simulink model "WelcomeBkwdStEnCtrl"  (R2018b)
settings: Solver=FixedStepDiscrete  StartTime=0.0  StopTime=10.0  FixedStep=0.01  RelTol=1e-3
undefined symbols (not defined in the file or in its folder): data, SecRwLtStBkReclnEn_Clear, SecRwLtStBkReclnEn_Set, SecRwLtStFwdBkwdEn_Clear, SecRwLtStFwdBkwdEn_Set, SecRwLtStHdrstFwdBkwdEn_Clear, SecRwLtStHdrstFwdBkwdEn_Set, SecRwLtStHdrstUpwdDnwdEn_Clear, SecRwLtStHdrstUpwdDnwdEn_Set, SecRwRtStBkReclnEn_Clear, SecRwRtStBkReclnEn_Set, SecRwRtStFwdBkwdEn_Clear, SecRwRtStFwdBkwdEn_Set, SecRwRtStHdrstFwdBkwdEn_Clear, SecRwRtStHdrstFwdBkwdEn_Set, SecRwRtStHdrstUpwdDnwdEn_Clear, SecRwRtStHdrstUpwdDnwdEn_Set
libraries: simulink x1
settings Model: ModifiedHistory=2023.8.1 V2.0.0 CR421790 增加模式21-26  Creator=sn2xws  LastModifiedBy=sn2xws
settings DataIOCC: SaveFormat=StructureWithTime
settings OptimizationCC: DefaultParameterBehavior=Inlined  EnhancedBackFolding=on  PassReuseOutputArgsAs=Individual arguments  ZeroExternalMemoryAtStartup=off  ZeroInternalMemoryAtStartup=off  OptimizeBlockOrder=speed  DifferentSizesBufferReuse=on  OptimizationCustomize=off
settings DebuggingCC: ParameterTunabilityLossMsg=error
settings SFSimCC: MATLABDynamicMemAlloc=off
settings RTWCC: SystemTargetFile=autosar.tlc  GenCodeOnly=on  TemplateMakefile=ert_default_tmf  Description=AUTOSAR  GenerateReport=on  IncludeHyperlinkInReport=on  LaunchReport=on  GenerateTraceInfo=on  GenerateTraceReport=on  GenerateTraceReportSl=on  GenerateTraceReportSf=on  GenerateTraceReportEml=on  GenerateCodeMetricsReport=on
settings CodeAppCC: ForceParamTrailComments=on  IgnoreCustomStorageClasses=off  OperatorAnnotations=on  SimulinkDataObjDesc=on  SFDataObjDesc=on  InsertBlockDesc=on
settings STFCustomTargetCC: TargetLangStandard=C99 (ISO)  MultiwordLength=256  ParMdlRefBuildCompliant=on  CompOptLevelCompliant=on  IncludeMdlTerminateFcn=off  CombineOutputUpdateFcns=on  SuppressErrorStatus=on  ERTCustomFileBanners=on  SupportNonFinite=off  SupportComplex=off  SupportContinuousTime=off  SupportNonInlinedSFcns=off  RemoveResetFunc=on  MATLABClassNameForMDSCustomization=Simulink.SoftwareTarget.ERTCustomization  AutosarCompliant=on  UseToolchainInfoCompliant=on  LookupTableObjectStructAxisOrder=2,1,3,4,...  LUTObjectStructOrderEvenSpacing=Size,Table,Breakpoints  SystemTargetFile=autosar.tlc
settings ERTTargetCC: TargetLangStandard=C99 (ISO)  ConcurrentExecutionCompliant=off  IncludeMdlTerminateFcn=off  SuppressErrorStatus=on  SupportNonFinite=off  SupportComplex=off  ModelStepFunctionPrototypeControlCompliant=off  CPPClassGenCompliant=off  AutosarCompliant=on  LookupTableObjectStructAxisOrder=2,1,3,4,...  LUTObjectStructOrderEvenSpacing=Size,Table,Breakpoints  InlinedParameterPlacement=NonHierarchical  ERTCustomFileTemplate=example_file_process.tlc  ERTFilePackagingFormat=Compact

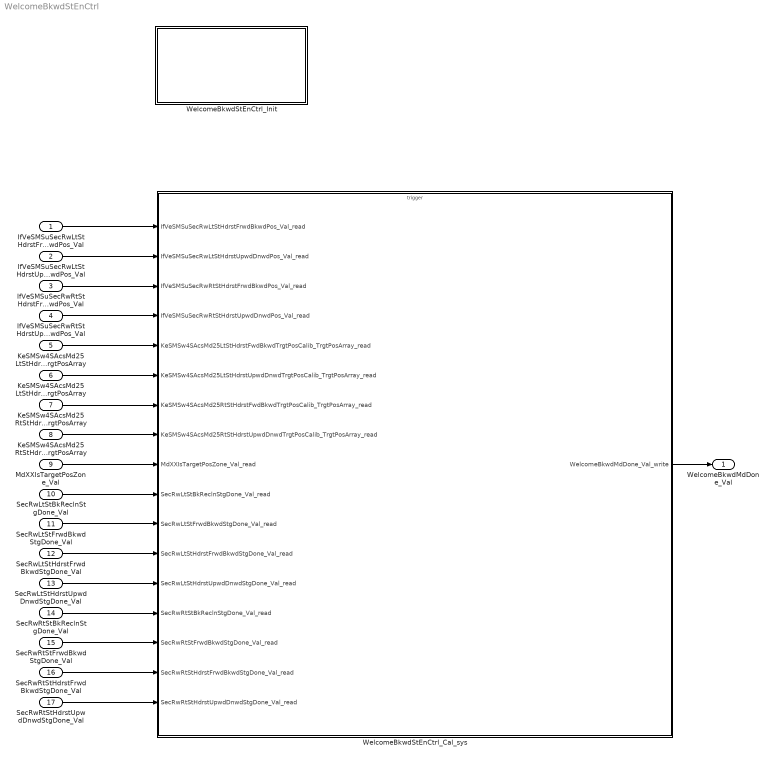
== system WelcomeBkwdStEnCtrl ==
  IfVeSMSuSecRwLtStHdrstFrwdBkwdPos_Val : Inport  OutDataTypeStr=uint16  PortDimensions=1
  IfVeSMSuSecRwLtStHdrstUpwdDnwdPos_Val : Inport  Port=2  OutDataTypeStr=uint16  PortDimensions=1
  IfVeSMSuSecRwRtStHdrstFrwdBkwdPos_Val : Inport  Port=3  OutDataTypeStr=uint16  PortDimensions=1
  IfVeSMSuSecRwRtStHdrstUpwdDnwdPos_Val : Inport  Port=4  OutDataTypeStr=uint16  PortDimensions=1
  KeSMSw4SAcsMd25LtStHdrstFwdBkwdTrgtPosCalib_TrgtPosArray : Inport  Description=|  Port=5  OutDataTypeStr=uint16  PortDimensions=3
      | 0:Pos
      | 1:Max
      | 2:Min
  KeSMSw4SAcsMd25LtStHdrstUpwdDnwdTrgtPosCalib_TrgtPosArray : Inport  Description=|  Port=6  OutDataTypeStr=uint16  PortDimensions=3
      | 0:Pos
      | 1:Max
      | 2:Min
  KeSMSw4SAcsMd25RtStHdrstFwdBkwdTrgtPosCalib_TrgtPosArray : Inport  Description=|  Port=7  OutDataTypeStr=uint16  PortDimensions=3
      | 0:Pos
      | 1:Max
      | 2:Min
  KeSMSw4SAcsMd25RtStHdrstUpwdDnwdTrgtPosCalib_TrgtPosArray : Inport  Description=|  Port=8  OutDataTypeStr=uint16  PortDimensions=3
      | 0:Pos
      | 1:Max
      | 2:Min
  MdXXIsTargetPosZone_Val : Inport  Port=9  OutDataTypeStr=uint32  PortDimensions=1
  SecRwLtStBkReclnStgDone_Val : Inport  Port=10  OutDataTypeStr=boolean  PortDimensions=1
  SecRwLtStFrwdBkwdStgDone_Val : Inport  Port=11  OutDataTypeStr=boolean  PortDimensions=1
  SecRwLtStHdrstFrwdBkwdStgDone_Val : Inport  Port=12  OutDataTypeStr=boolean  PortDimensions=1
  SecRwLtStHdrstUpwdDnwdStgDone_Val : Inport  Port=13  OutDataTypeStr=boolean  PortDimensions=1
  SecRwRtStBkReclnStgDone_Val : Inport  Port=14  OutDataTypeStr=boolean  PortDimensions=1
  SecRwRtStFrwdBkwdStgDone_Val : Inport  Port=15  OutDataTypeStr=boolean  PortDimensions=1
  SecRwRtStHdrstFrwdBkwdStgDone_Val : Inport  Port=16  OutDataTypeStr=boolean  PortDimensions=1
  SecRwRtStHdrstUpwdDnwdStgDone_Val : Inport  Port=17  OutDataTypeStr=boolean  PortDimensions=1
  WelcomeBkwdStEnCtrl_Cal_sys : Subsystem
  WelcomeBkwdStEnCtrl_Init : Subsystem
  WelcomeBkwdMdDone_Val : Outport  OutDataTypeStr=uint8  PortDimensions=1
  wires:
  IfVeSMSuSecRwLtStHdrstFrwdBkwdPos_Val/1 -> WelcomeBkwdStEnCtrl_Cal_sys/1(IfVeSMSuSecRwLtStHdrstFrwdBkwdPos_Val_read)
  IfVeSMSuSecRwLtStHdrstUpwdDnwdPos_Val/1 -> WelcomeBkwdStEnCtrl_Cal_sys/2(IfVeSMSuSecRwLtStHdrstUpwdDnwdPos_Val_read)
  IfVeSMSuSecRwRtStHdrstFrwdBkwdPos_Val/1 -> WelcomeBkwdStEnCtrl_Cal_sys/3(IfVeSMSuSecRwRtStHdrstFrwdBkwdPos_Val_read)
  IfVeSMSuSecRwRtStHdrstUpwdDnwdPos_Val/1 -> WelcomeBkwdStEnCtrl_Cal_sys/4(IfVeSMSuSecRwRtStHdrstUpwdDnwdPos_Val_read)
  KeSMSw4SAcsMd25LtStHdrstFwdBkwdTrgtPosCalib_TrgtPosArray/1 -> WelcomeBkwdStEnCtrl_Cal_sys/5(KeSMSw4SAcsMd25LtStHdrstFwdBkwdTrgtPosCalib_TrgtPosArray_read)
  KeSMSw4SAcsMd25LtStHdrstUpwdDnwdTrgtPosCalib_TrgtPosArray/1 -> WelcomeBkwdStEnCtrl_Cal_sys/6(KeSMSw4SAcsMd25LtStHdrstUpwdDnwdTrgtPosCalib_TrgtPosArray_read)
  KeSMSw4SAcsMd25RtStHdrstFwdBkwdTrgtPosCalib_TrgtPosArray/1 -> WelcomeBkwdStEnCtrl_Cal_sys/7(KeSMSw4SAcsMd25RtStHdrstFwdBkwdTrgtPosCalib_TrgtPosArray_read)
  KeSMSw4SAcsMd25RtStHdrstUpwdDnwdTrgtPosCalib_TrgtPosArray/1 -> WelcomeBkwdStEnCtrl_Cal_sys/8(KeSMSw4SAcsMd25RtStHdrstUpwdDnwdTrgtPosCalib_TrgtPosArray_read)
  MdXXIsTargetPosZone_Val/1 -> WelcomeBkwdStEnCtrl_Cal_sys/9(MdXXIsTargetPosZone_Val_read)
  SecRwLtStBkReclnStgDone_Val/1 -> WelcomeBkwdStEnCtrl_Cal_sys/10(SecRwLtStBkReclnStgDone_Val_read)
  SecRwLtStFrwdBkwdStgDone_Val/1 -> WelcomeBkwdStEnCtrl_Cal_sys/11(SecRwLtStFrwdBkwdStgDone_Val_read)
  SecRwLtStHdrstFrwdBkwdStgDone_Val/1 -> WelcomeBkwdStEnCtrl_Cal_sys/12(SecRwLtStHdrstFrwdBkwdStgDone_Val_read)
  SecRwLtStHdrstUpwdDnwdStgDone_Val/1 -> WelcomeBkwdStEnCtrl_Cal_sys/13(SecRwLtStHdrstUpwdDnwdStgDone_Val_read)
  SecRwRtStBkReclnStgDone_Val/1 -> WelcomeBkwdStEnCtrl_Cal_sys/14(SecRwRtStBkReclnStgDone_Val_read)
  SecRwRtStFrwdBkwdStgDone_Val/1 -> WelcomeBkwdStEnCtrl_Cal_sys/15(SecRwRtStFrwdBkwdStgDone_Val_read)
  SecRwRtStHdrstFrwdBkwdStgDone_Val/1 -> WelcomeBkwdStEnCtrl_Cal_sys/16(SecRwRtStHdrstFrwdBkwdStgDone_Val_read)
  SecRwRtStHdrstUpwdDnwdStgDone_Val/1 -> WelcomeBkwdStEnCtrl_Cal_sys/17(SecRwRtStHdrstUpwdDnwdStgDone_Val_read)
  WelcomeBkwdStEnCtrl_Cal_sys/1(WelcomeBkwdMdDone_Val_write) -> WelcomeBkwdMdDone_Val/1

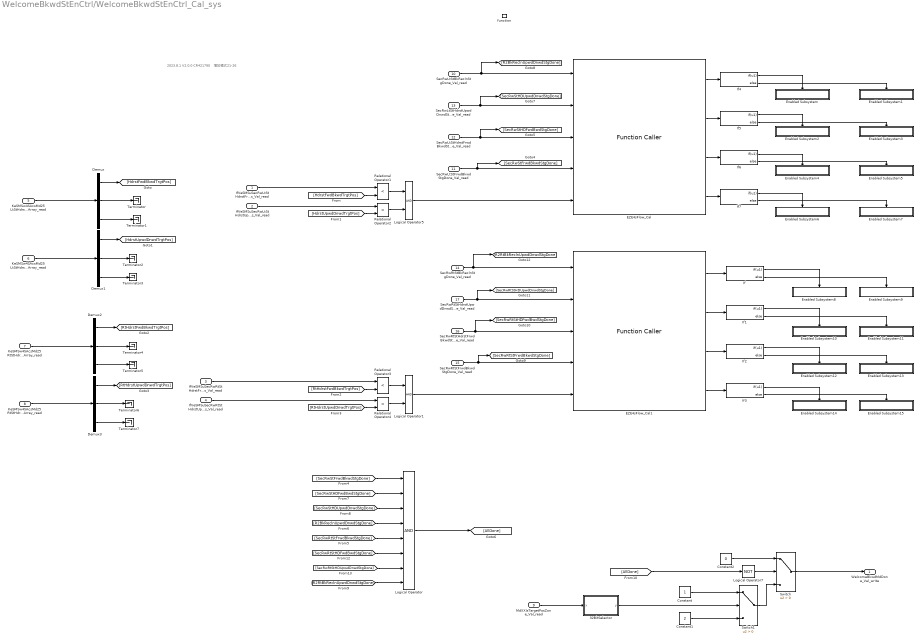
== system WelcomeBkwdStEnCtrl/WelcomeBkwdStEnCtrl_Cal_sys ==
  note: 2023.8.1 V2.0.0 CR421790 增加模式21-26
  IfVeSMSuSecRwLtStHdrstFrwdBkwdPos_Val_read : Inport
  IfVeSMSuSecRwLtStHdrstUpwdDnwdPos_Val_read : Inport  Port=2
  IfVeSMSuSecRwRtStHdrstFrwdBkwdPos_Val_read : Inport  Port=3
  IfVeSMSuSecRwRtStHdrstUpwdDnwdPos_Val_read : Inport  Port=4
  KeSMSw4SAcsMd25LtStHdrstFwdBkwdTrgtPosCalib_TrgtPosArray_read : Inport  Port=5
  KeSMSw4SAcsMd25LtStHdrstUpwdDnwdTrgtPosCalib_TrgtPosArray_read : Inport  Port=6
  KeSMSw4SAcsMd25RtStHdrstFwdBkwdTrgtPosCalib_TrgtPosArray_read : Inport  Port=7
  KeSMSw4SAcsMd25RtStHdrstUpwdDnwdTrgtPosCalib_TrgtPosArray_read : Inport  Port=8
  MdXXIsTargetPosZone_Val_read : Inport  Port=9
  SecRwLtStBkReclnStgDone_Val_read : Inport  Port=10
  SecRwLtStFrwdBkwdStgDone_Val_read : Inport  Port=11
  SecRwLtStHdrstFrwdBkwdStgDone_Val_read : Inport  Port=12
  SecRwLtStHdrstUpwdDnwdStgDone_Val_read : Inport  Port=13
  SecRwRtStBkReclnStgDone_Val_read : Inport  Port=14
  SecRwRtStFrwdBkwdStgDone_Val_read : Inport  Port=15
  SecRwRtStHdrstFrwdBkwdStgDone_Val_read : Inport  Port=16
  SecRwRtStHdrstUpwdDnwdStgDone_Val_read : Inport  Port=17
  function : TriggerPort  TriggerType=function-call  IsSimulinkFunction=on  FunctionName=WelcomeBkwdStEnCtrl_Cal  VariantControl=(inherit)
  32BitSelector : Subsystem  mask(32 Bit Selector){BitNum=24}
      mask prompts: BitNum "Select Bit Number"
      mask help: Allows selection of a particular bit (0-31) out of a packed word up to 32 bits long. Output will be true if the bit number selected via the mask parameter is equal to one.
      mask TypeOptions BitNum: 0 | 1 | 2 | 3 | 4 | 5 | 6 | 7 | 8 | 9 | 10 | 11 | 12 | 13 | 14 | 15 | 16 | 17 | 18 | 19 | 20 | 21 | 22 | 23 | 24 | 25 | 26 | 27 | 28 | 29 | 30 | 31
      mask Display:
      | text(0.5, 0.8,'BIT','horizontalAlignment','center')
      | text(0.5, 0.5,'SELECTOR','horizontalAlignment','center')
      | text(0.5, 0.2,['-- Bit ',char(get_param(gcb,'BitNum')),' --'],'horizontalAlignment','center')
  Constant : Constant  OutDataTypeStr=uint8
  Constant1 : Constant  Value=2  OutDataTypeStr=uint8
  Constant2 : Constant  Value=0  OutDataTypeStr=uint8
  Demux{,1..3} (4 alike) : Demux  Outputs=3
  EZE4sFlow_Cal : FunctionCaller  FunctionPrototype=[BkReclnEn,HdrstUpwdEn,HdrstFrwdEn,SecRwStFrwdBkwdEn] = EZE4sFlow_Cal(BkReclnStgDone,HdrstUpwdDnwdStgDone,HdrstFrwdBkwdStgDone,SecRwStFrwdBkwdStgDone,Chkhdflg)  InputArgumentSpecifications=boolean(true), boolean(true), boolean(true), boolean(true), boolean(true)  OutputArgumentSpecifications=boolean(true), boolean(true), boolean(true), boolean(true)
  EZE4sFlow_Cal1 : FunctionCaller  FunctionPrototype=[BkReclnEn,HdrstUpwdEn,HdrstFrwdEn,SecRwStFrwdBkwdEn] = EZE4sFlow_Cal(BkReclnStgDone,HdrstUpwdDnwdStgDone,HdrstFrwdBkwdStgDone,SecRwStFrwdBkwdStgDone,Chkhdflg)  InputArgumentSpecifications=boolean(true), boolean(true), boolean(true), boolean(true), boolean(true)  OutputArgumentSpecifications=boolean(true), boolean(true), boolean(true), boolean(true)
  Enabled Subsystem : Subsystem  TreatAsAtomicUnit=on
  Enabled Subsystem1 : Subsystem  TreatAsAtomicUnit=on
  Enabled Subsystem10 : Subsystem  TreatAsAtomicUnit=on
  Enabled Subsystem11 : Subsystem  TreatAsAtomicUnit=on
  Enabled Subsystem12 : Subsystem  TreatAsAtomicUnit=on
  Enabled Subsystem13 : Subsystem  TreatAsAtomicUnit=on
  Enabled Subsystem14 : Subsystem  TreatAsAtomicUnit=on
  Enabled Subsystem15 : Subsystem  TreatAsAtomicUnit=on
  Enabled Subsystem2 : Subsystem  TreatAsAtomicUnit=on
  Enabled Subsystem3 : Subsystem  TreatAsAtomicUnit=on
  Enabled Subsystem4 : Subsystem  TreatAsAtomicUnit=on
  Enabled Subsystem5 : Subsystem  TreatAsAtomicUnit=on
  Enabled Subsystem6 : Subsystem  TreatAsAtomicUnit=on
  Enabled Subsystem7 : Subsystem  TreatAsAtomicUnit=on
  Enabled Subsystem8 : Subsystem  TreatAsAtomicUnit=on
  Enabled Subsystem9 : Subsystem  TreatAsAtomicUnit=on
  If{,1..7} (8 alike) : If  IfExpression=u1
  Logical Operator : Logic  Inputs=8  AllPortsSameDT=off  OutDataTypeStr=boolean
  Logical Operator1 : Logic  AllPortsSameDT=off  OutDataTypeStr=boolean
  Logical Operator5 : Logic  AllPortsSameDT=off  OutDataTypeStr=boolean
  Logical Operator7 : Logic  Operator=NOT  AllPortsSameDT=off  OutDataTypeStr=boolean
  Relational Operator{1..4} (4 alike) : RelationalOperator  Operator=<  OutDataTypeStr=boolean  RndMeth=Simplest
  Switch : Switch  Criteria=u2 > Threshold
  Switch1 : Switch  Criteria=u2 > Threshold
  Terminator{,1..7} (8 alike) : Terminator
  WelcomeBkwdMdDone_Val_write : Outport
      settings: EnsureOutportIsVirtual=on
  wires:
  SecRwLtStFrwdBkwdStgDone_Val_read/1 -> EZE4sFlow_Cal/4, [SecRwStFrwdBkwdStgDone]
  SecRwLtStHdrstFrwdBkwdStgDone_Val_read/1 -> [SecRwStHDFwdBwdStgDone], EZE4sFlow_Cal/3
  SecRwLtStHdrstUpwdDnwdStgDone_Val_read/1 -> [SecRwStHDUpwdDnwdStgDone], EZE4sFlow_Cal/2
  SecRwLtStBkReclnStgDone_Val_read/1 -> [R2BkReclnUpwdDnwdStgDone], EZE4sFlow_Cal/1
  SecRwRtStBkReclnStgDone_Val_read/1 -> [R2RtBkReclnUpwdDnwdStgDone], EZE4sFlow_Cal1/1
  SecRwRtStFrwdBkwdStgDone_Val_read/1 -> [SecRwRtStFrwdBkwdStgDone], EZE4sFlow_Cal1/4
  SecRwRtStHdrstFrwdBkwdStgDone_Val_read/1 -> [SecRwRtStHDFwdBwdStgDone], EZE4sFlow_Cal1/3
  SecRwRtStHdrstUpwdDnwdStgDone_Val_read/1 -> [SecRwRtStHDUpwdDnwdStgDone], EZE4sFlow_Cal1/2
  [HdrstFwdBkwdTrgtPos] -> Relational Operator1/2
  IfVeSMSuSecRwLtStHdrstFrwdBkwdPos_Val_read/1 -> Relational Operator1/1
  IfVeSMSuSecRwLtStHdrstUpwdDnwdPos_Val_read/1 -> Relational Operator2/1
  Relational Operator2/1 -> Logical Operator5/2
  [HdrstUpwdDnwdTrgtPos] -> Relational Operator2/2
  Relational Operator1/1 -> Logical Operator5/1
  Logical Operator5/1 -> EZE4sFlow_Cal/5
  Logical Operator1/1 -> EZE4sFlow_Cal1/5
  Relational Operator3/1 -> Logical Operator1/1
  [RtHdrstUpwdDnwdTrgtPos] -> Relational Operator4/2
  Relational Operator4/1 -> Logical Operator1/2
  IfVeSMSuSecRwRtStHdrstUpwdDnwdPos_Val_read/1 -> Relational Operator4/1
  IfVeSMSuSecRwRtStHdrstFrwdBkwdPos_Val_read/1 -> Relational Operator3/1
  [RtHdrstFwdBkwdTrgtPos] -> Relational Operator3/2
  Demux1/1 -> [HdrstUpwdDnwdTrgtPos]
  KeSMSw4SAcsMd25LtStHdrstFwdBkwdTrgtPosCalib_TrgtPosArray_read/1 -> Demux/1
  Demux1/3 -> Terminator3/1
  Demux/1 -> [HdrstFwdBkwdTrgtPos]
  Demux/2 -> Terminator/1
  KeSMSw4SAcsMd25LtStHdrstUpwdDnwdTrgtPosCalib_TrgtPosArray_read/1 -> Demux1/1
  Demux1/2 -> Terminator2/1
  Demux/3 -> Terminator1/1
  Demux2/3 -> Terminator5/1
  Demux3/2 -> Terminator6/1
  KeSMSw4SAcsMd25RtStHdrstUpwdDnwdTrgtPosCalib_TrgtPosArray_read/1 -> Demux3/1
  Demux2/2 -> Terminator4/1
  Demux2/1 -> [RtHdrstFwdBkwdTrgtPos]
  Demux3/3 -> Terminator7/1
  KeSMSw4SAcsMd25RtStHdrstFwdBkwdTrgtPosCalib_TrgtPosArray_read/1 -> Demux2/1
  Demux3/1 -> [RtHdrstUpwdDnwdTrgtPos]
  [R2BkReclnUpwdDnwdStgDone] -> Logical Operator/4
  Logical Operator/1 -> [AllDone]
  [SecRwStFrwdBkwdStgDone] -> Logical Operator/1
  [SecRwStHDUpwdDnwdStgDone] -> Logical Operator/3
  [SecRwStHDFwdBwdStgDone] -> Logical Operator/2
  Switch1/1 -> Switch/3
  MdXXIsTargetPosZone_Val_read/1 -> 32BitSelector/1(x)
  Switch/1 -> WelcomeBkwdMdDone_Val_write/1
  [SecRwRtStHDFwdBwdStgDone] -> Logical Operator/6
  [SecRwRtStHDUpwdDnwdStgDone] -> Logical Operator/7
  [SecRwRtStFrwdBkwdStgDone] -> Logical Operator/5
  [R2RtBkReclnUpwdDnwdStgDone] -> Logical Operator/8
  EZE4sFlow_Cal1/1 -> If/1
  If/1 -> Enabled Subsystem8/Action
  If/2 -> Enabled Subsystem9/Action
  EZE4sFlow_Cal1/2 -> If1/1
  EZE4sFlow_Cal1/4 -> If3/1
  EZE4sFlow_Cal1/3 -> If2/1
  If1/1 -> Enabled Subsystem10/Action
  If1/2 -> Enabled Subsystem11/Action
  If2/1 -> Enabled Subsystem12/Action
  If2/2 -> Enabled Subsystem13/Action
  If3/1 -> Enabled Subsystem14/Action
  If3/2 -> Enabled Subsystem15/Action
  EZE4sFlow_Cal/1 -> If4/1
  EZE4sFlow_Cal/2 -> If5/1
  EZE4sFlow_Cal/3 -> If6/1
  EZE4sFlow_Cal/4 -> If7/1
  If4/1 -> Enabled Subsystem/Action
  If4/2 -> Enabled Subsystem1/Action
  If5/1 -> Enabled Subsystem2/Action
  If5/2 -> Enabled Subsystem3/Action
  If6/1 -> Enabled Subsystem4/Action
  If6/2 -> Enabled Subsystem5/Action
  If7/1 -> Enabled Subsystem6/Action
  If7/2 -> Enabled Subsystem7/Action
  Constant2/1 -> Switch/1
  Constant1/1 -> Switch1/3
  Constant/1 -> Switch1/1
  [AllDone] -> Logical Operator7/1
  Logical Operator7/1 -> Switch/2
  32BitSelector/1(y) -> Switch1/2

== system WelcomeBkwdStEnCtrl/WelcomeBkwdStEnCtrl_Init ==
  Event Listener : EventListener  EventName=reset

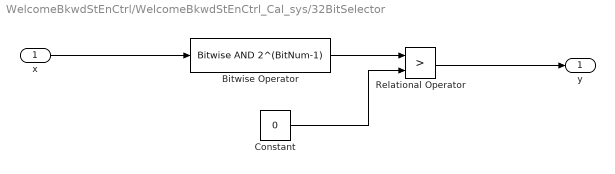
== system WelcomeBkwdStEnCtrl/WelcomeBkwdStEnCtrl_Cal_sys/32BitSelector ==
  x : Inport
  Bitwise Operator : simulink/Logic and Bit Operations/Bitwise Operator  logicop=AND  UseBitMask=on  BitMask=2^(BitNum-1)  BitMaskRealWorld=Stored Integer
  Constant : Constant  Value=0  OutDataTypeStr=uint32
  Relational Operator : RelationalOperator  Operator=>  OutDataTypeStr=boolean  RndMeth=Simplest
  y : Outport
  wires:
  Relational Operator/1 -> y/1
  Constant/1 -> Relational Operator/2
  x/1 -> Bitwise Operator/1
  Bitwise Operator/1 -> Relational Operator/1

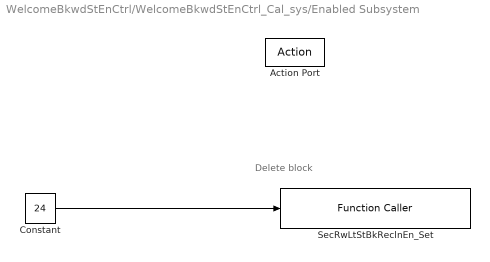
== system WelcomeBkwdStEnCtrl/WelcomeBkwdStEnCtrl_Cal_sys/Enabled Subsystem ==
  note: Delete block
  Action Port : ActionPort  ActionType=then
  Constant : Constant  Value=24  OutDataTypeStr=uint8
  SecRwLtStBkReclnEn_Set : FunctionCaller  FunctionPrototype=SecRwLtStBkReclnEn_Set(data)  InputArgumentSpecifications=uint8(1)
  wires:
  Constant/1 -> SecRwLtStBkReclnEn_Set/1

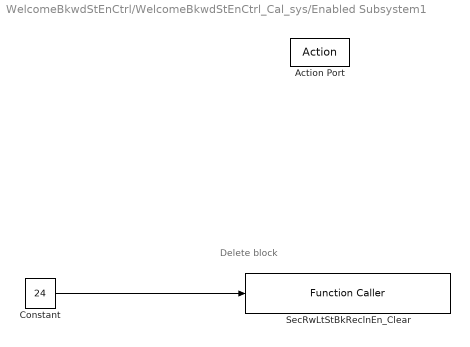
== system WelcomeBkwdStEnCtrl/WelcomeBkwdStEnCtrl_Cal_sys/Enabled Subsystem1 ==
  note: Delete block
  Action Port : ActionPort  ActionType=else
  Constant : Constant  Value=24  OutDataTypeStr=uint8
  SecRwLtStBkReclnEn_Clear : FunctionCaller  FunctionPrototype=SecRwLtStBkReclnEn_Clear(data)  InputArgumentSpecifications=uint8(1)
  wires:
  Constant/1 -> SecRwLtStBkReclnEn_Clear/1

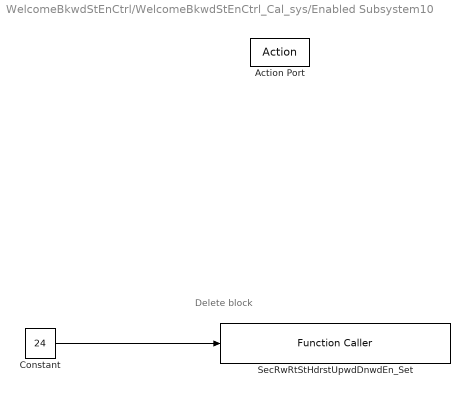
== system WelcomeBkwdStEnCtrl/WelcomeBkwdStEnCtrl_Cal_sys/Enabled Subsystem10 ==
  note: Delete block
  Action Port : ActionPort  ActionType=then
  Constant : Constant  Value=24  OutDataTypeStr=uint8
  SecRwRtStHdrstUpwdDnwdEn_Set : FunctionCaller  FunctionPrototype=SecRwRtStHdrstUpwdDnwdEn_Set(data)  InputArgumentSpecifications=uint8(1)
  wires:
  Constant/1 -> SecRwRtStHdrstUpwdDnwdEn_Set/1

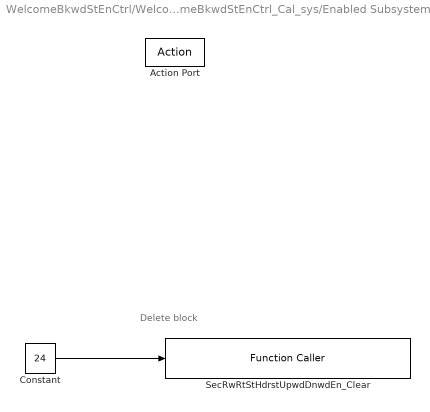
== system WelcomeBkwdStEnCtrl/WelcomeBkwdStEnCtrl_Cal_sys/Enabled Subsystem11 ==
  note: Delete block
  Action Port : ActionPort  ActionType=else
  Constant : Constant  Value=24  OutDataTypeStr=uint8
  SecRwRtStHdrstUpwdDnwdEn_Clear : FunctionCaller  FunctionPrototype=SecRwRtStHdrstUpwdDnwdEn_Clear(data)  InputArgumentSpecifications=uint8(1)
  wires:
  Constant/1 -> SecRwRtStHdrstUpwdDnwdEn_Clear/1

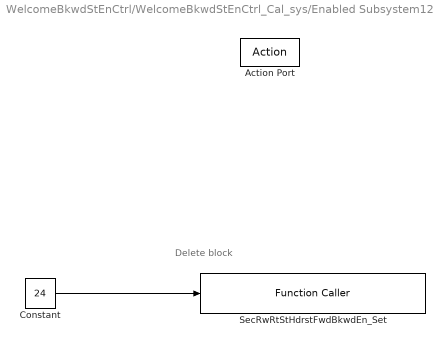
== system WelcomeBkwdStEnCtrl/WelcomeBkwdStEnCtrl_Cal_sys/Enabled Subsystem12 ==
  note: Delete block
  Action Port : ActionPort  ActionType=then
  Constant : Constant  Value=24  OutDataTypeStr=uint8
  SecRwRtStHdrstFwdBkwdEn_Set : FunctionCaller  FunctionPrototype=SecRwRtStHdrstFwdBkwdEn_Set(data)  InputArgumentSpecifications=uint8(1)
  wires:
  Constant/1 -> SecRwRtStHdrstFwdBkwdEn_Set/1

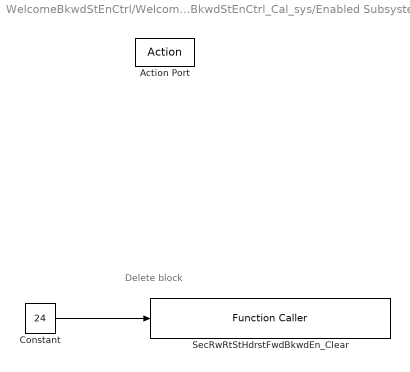
== system WelcomeBkwdStEnCtrl/WelcomeBkwdStEnCtrl_Cal_sys/Enabled Subsystem13 ==
  note: Delete block
  Action Port : ActionPort  ActionType=else
  Constant : Constant  Value=24  OutDataTypeStr=uint8
  SecRwRtStHdrstFwdBkwdEn_Clear : FunctionCaller  FunctionPrototype=SecRwRtStHdrstFwdBkwdEn_Clear(data)  InputArgumentSpecifications=uint8(1)
  wires:
  Constant/1 -> SecRwRtStHdrstFwdBkwdEn_Clear/1

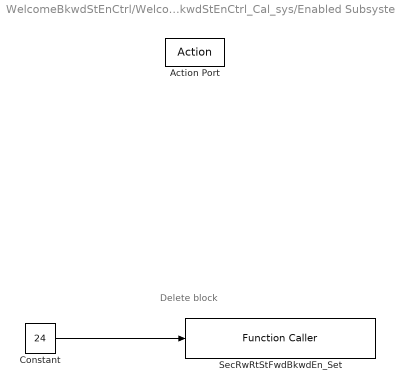
== system WelcomeBkwdStEnCtrl/WelcomeBkwdStEnCtrl_Cal_sys/Enabled Subsystem14 ==
  note: Delete block
  Action Port : ActionPort  ActionType=then
  Constant : Constant  Value=24  OutDataTypeStr=uint8
  SecRwRtStFwdBkwdEn_Set : FunctionCaller  FunctionPrototype=SecRwRtStFwdBkwdEn_Set(data)  InputArgumentSpecifications=uint8(1)
  wires:
  Constant/1 -> SecRwRtStFwdBkwdEn_Set/1

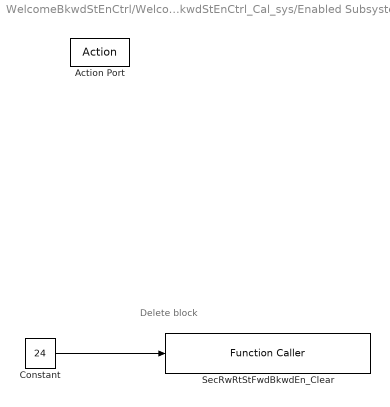
== system WelcomeBkwdStEnCtrl/WelcomeBkwdStEnCtrl_Cal_sys/Enabled Subsystem15 ==
  note: Delete block
  Action Port : ActionPort  ActionType=else
  Constant : Constant  Value=24  OutDataTypeStr=uint8
  SecRwRtStFwdBkwdEn_Clear : FunctionCaller  FunctionPrototype=SecRwRtStFwdBkwdEn_Clear(data)  InputArgumentSpecifications=uint8(1)
  wires:
  Constant/1 -> SecRwRtStFwdBkwdEn_Clear/1

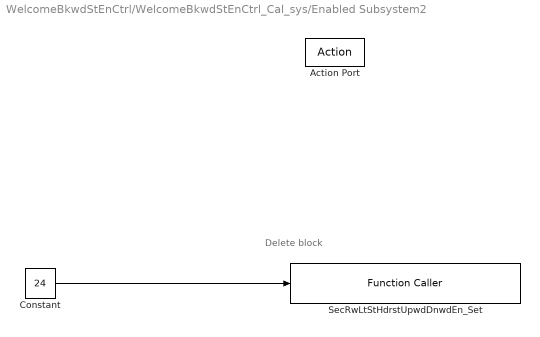
== system WelcomeBkwdStEnCtrl/WelcomeBkwdStEnCtrl_Cal_sys/Enabled Subsystem2 ==
  note: Delete block
  Action Port : ActionPort  ActionType=then
  Constant : Constant  Value=24  OutDataTypeStr=uint8
  SecRwLtStHdrstUpwdDnwdEn_Set : FunctionCaller  FunctionPrototype=SecRwLtStHdrstUpwdDnwdEn_Set(data)  InputArgumentSpecifications=uint8(1)
  wires:
  Constant/1 -> SecRwLtStHdrstUpwdDnwdEn_Set/1

== system WelcomeBkwdStEnCtrl/WelcomeBkwdStEnCtrl_Cal_sys/Enabled Subsystem3 ==
  note: Delete block
  Action Port : ActionPort  ActionType=else
  Constant : Constant  Value=24  OutDataTypeStr=uint8
  SecRwLtStHdrstUpwdDnwdEn_Clear : FunctionCaller  FunctionPrototype=SecRwLtStHdrstUpwdDnwdEn_Clear(data)  InputArgumentSpecifications=uint8(1)
  wires:
  Constant/1 -> SecRwLtStHdrstUpwdDnwdEn_Clear/1

== system WelcomeBkwdStEnCtrl/WelcomeBkwdStEnCtrl_Cal_sys/Enabled Subsystem4 ==
  note: Delete block
  Action Port : ActionPort  ActionType=then
  Constant : Constant  Value=24  OutDataTypeStr=uint8
  SecRwLtStHdrstFwdBkwdEn_Set : FunctionCaller  FunctionPrototype=SecRwLtStHdrstFwdBkwdEn_Set(data)  InputArgumentSpecifications=uint8(1)
  wires:
  Constant/1 -> SecRwLtStHdrstFwdBkwdEn_Set/1

== system WelcomeBkwdStEnCtrl/WelcomeBkwdStEnCtrl_Cal_sys/Enabled Subsystem5 ==
  note: Delete block
  Action Port : ActionPort  ActionType=else
  Constant : Constant  Value=24  OutDataTypeStr=uint8
  SecRwLtStHdrstFwdBkwdEn_Clear : FunctionCaller  FunctionPrototype=SecRwLtStHdrstFwdBkwdEn_Clear(data)  InputArgumentSpecifications=uint8(1)
  wires:
  Constant/1 -> SecRwLtStHdrstFwdBkwdEn_Clear/1

== system WelcomeBkwdStEnCtrl/WelcomeBkwdStEnCtrl_Cal_sys/Enabled Subsystem6 ==
  note: Delete block
  Action Port : ActionPort  ActionType=then
  Constant : Constant  Value=24  OutDataTypeStr=uint8
  SecRwLtStFwdBkwdEn_Set : FunctionCaller  FunctionPrototype=SecRwLtStFwdBkwdEn_Set(data)  InputArgumentSpecifications=uint8(1)
  wires:
  Constant/1 -> SecRwLtStFwdBkwdEn_Set/1

== system WelcomeBkwdStEnCtrl/WelcomeBkwdStEnCtrl_Cal_sys/Enabled Subsystem7 ==
  note: Delete block
  Action Port : ActionPort  ActionType=else
  Constant : Constant  Value=24  OutDataTypeStr=uint8
  SecRwLtStFwdBkwdEn_Clear : FunctionCaller  FunctionPrototype=SecRwLtStFwdBkwdEn_Clear(data)  InputArgumentSpecifications=uint8(1)
  wires:
  Constant/1 -> SecRwLtStFwdBkwdEn_Clear/1

== system WelcomeBkwdStEnCtrl/WelcomeBkwdStEnCtrl_Cal_sys/Enabled Subsystem8 ==
  note: Delete block
  Action Port : ActionPort  ActionType=then
  Constant : Constant  Value=24  OutDataTypeStr=uint8
  SecRwRtStBkReclnEn_Set : FunctionCaller  FunctionPrototype=SecRwRtStBkReclnEn_Set(data)  InputArgumentSpecifications=uint8(1)
  wires:
  Constant/1 -> SecRwRtStBkReclnEn_Set/1

== system WelcomeBkwdStEnCtrl/WelcomeBkwdStEnCtrl_Cal_sys/Enabled Subsystem9 ==
  note: Delete block
  Action Port : ActionPort  ActionType=else
  Constant : Constant  Value=24  OutDataTypeStr=uint8
  SecRwRtStBkReclnEn_Clear : FunctionCaller  FunctionPrototype=SecRwRtStBkReclnEn_Clear(data)  InputArgumentSpecifications=uint8(1)
  wires:
  Constant/1 -> SecRwRtStBkReclnEn_Clear/1
